simulink model "S_waage4"  (Simulink 2.00)
settings: Solver=ode15s  StartTime=0.0  StopTime=0.25  FixedStep=1e-4  MaxStep=1e-4  RelTol=1e-3  AbsTol=1e-6
values from neighbouring files (symbols this model uses):
  D = my_sys1.d    [ncd_estim1.m]    (also in ncd_estim_1.mat = 0; ncd_kalm1.m; ncd_kalm2.m; ncd_kalm_1.mat = 0)
  g = 9.8    [ident21.mat]    (also in torce11.m = 9.81; torcell.mat = 9.81; waag11.m = 9.81; waag11.mat = 9.81)
  kg = 5    [waag11.m]    (also in waag11.mat; waage2.m; waage3.m)
  kr = kr    (= 1000)    [waage3.m]
  ks = 200    [waag11.m]    (also in waag11.mat; waage2.m; waage3.m = 300)
  L = place(A, B, p)'    [ncd_estim1.m]    (also in ncd_estim_1.mat = [29.04 93.6748 304.13176 464.47352 317.56952 149.5392]; ncd_kalm_2.mat = [29.04 93.6748 304.13176 464.47352 317.56952 149.5392]; torce11.m = axis; torcell.mat = [0 100 0 3])
  mw = 0.1    [waag11.m]    (also in waag11.mat; waage2.m; waage3.m = 0.5)
  mx = 5    [waag11.m]    (also in waag11.mat; waage2.m; waage3.m)
  pr2 = ',num2str(pr2),                '    [waage3.m]
  pr3 = ',num2str(pr3)])    [waage3.m]
  R = 1    [ncd_estim1.m]    (also in ncd_estim_1.mat; ncd_kalm1.m; ncd_kalm2.m; ncd_kalm_1.mat)
  r = 0.0003    [ident21.mat]    (also in waag11.m = 100; waag11.mat = 100; waage2.m = 100; waage3.m = 100)
  zr1 = ',num2str(zr1),                '    [waage3.m]
  zr2 = ',num2str(zr2),                '    [waage3.m]
  zr3 = ',num2str(zr2),                '    [waage3.m]
settings Model: SaveTime=off  SaveOutput=off  ConsistencyChecking=off

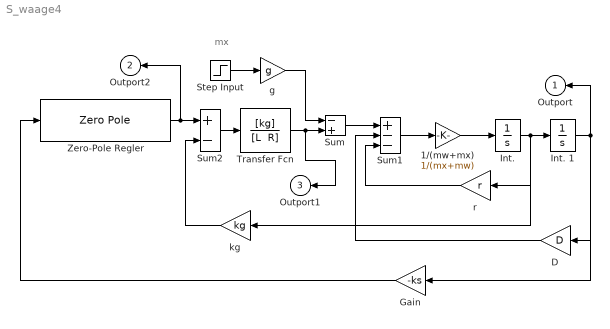
== system S_waage4 ==
  note: mx
  1/(mw+mx) : Gain  Gain=1/(mx+mw)
  D : Gain  Orientation=left  Gain=D
  Gain : Gain  Orientation=left  Gain=-ks
  Int. : Integrator  ExternalReset=none  InitialConditionSource=internal  InitialCondition=0  LimitOutput=off  UpperSaturationLimit=inf  LowerSaturationLimit=-inf  ShowSaturationPort=off  ShowStatePort=off  AbsoluteTolerance=auto
  Int. 1 : Integrator  ExternalReset=none  InitialConditionSource=internal  InitialCondition=0  LimitOutput=off  UpperSaturationLimit=inf  LowerSaturationLimit=-inf  ShowSaturationPort=off  ShowStatePort=off  AbsoluteTolerance=auto
  Step Input : Step  Time=0  Before=0  After=mx
  Sum : Sum  Inputs=-+
  Sum1 : Sum  Inputs=+--
  Sum2 : Sum  Inputs=+-
  Transfer Fcn : TransferFcn  Numerator=[kg]  Denominator="[L  R]"
  Zero-Pole Regler : ZeroPole  Zeros=[zr1; zr2; zr3]  Poles=[0; pr2; pr3]  Gain=[kr]
  g : Gain  Gain=g
  kg : Gain  Orientation=left  Gain=kg
  r : Gain  Orientation=left  Gain=r
  Outport : Outport  Orientation=left  Port=1  InitialOutput=0
  Outport2 : Outport  Orientation=left  Port=2  InitialOutput=0
  Outport1 : Outport  Orientation=left  Port=3  InitialOutput=0
  wires:
  Zero-Pole Regler/1 -> Outport2/1, Sum2/1
  Transfer Fcn/1 -> Outport1/1, Sum/2
  kg/1 -> Sum2/2
  Gain/1 -> Zero-Pole Regler/1
  Int. 1/1 -> Gain/1, Outport/1, D/1
  Sum2/1 -> Transfer Fcn/1
  r/1 -> Sum1/3
  Int./1 -> kg/1, r/1, Int. 1/1
  D/1 -> Sum1/2
  1/(mw+mx)/1 -> Int./1
  Sum1/1 -> 1/(mw+mx)/1
  Sum/1 -> Sum1/1
  g/1 -> Sum/1
  Step Input/1 -> g/1
